simulink model "zad_5_sch_dyskretny"  (R2022b)
settings: Solver=FixedStepAuto  StartTime=0.0  StopTime=1  FixedStep=0.0001  RelTol=1e-3
values from neighbouring files (symbols this model uses):
  A = [0 1 0; a21 0 a23; a31 0 a33]    [zad_5.m]
  B = [0 0; 0 g; b31 0]    [zad_5.m]
  C = [1 0 0]    [zad_5.m]
  Kx = -acker(A, B(:,1), -sKx)    [zad_5.m]
  u0 = -(a31*x1+a33*x3)/b31    [zad_5.m]
  x1 = .003    (= 0.003)    [zad_5.m]
  x2 = 0    [zad_5.m]
  x3 = -(a21*x1+g)/a23    [zad_5.m]
  xd = d-bd    (= 0.0192)    [zad_5.m]
settings Model: Creator=MPatr  LastModifiedBy=AgraWoodAdmin
settings SolverCC: AlgebraicLoopSolver=TrustRegion
settings DebuggingCC: ArithmeticOperatorsInVariantConditions=warning
settings SFSimCC: CustomCodeUndefinedFunction=UseInterfaceOnly

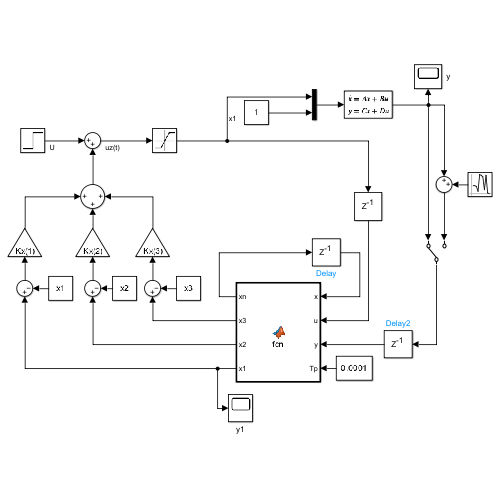
[thumbnail: Simulink's stored preview of the top-level diagram]
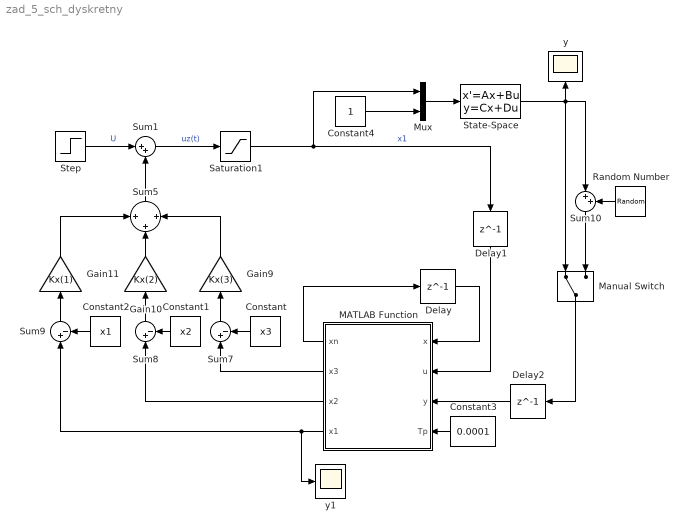
== system zad_5_sch_dyskretny ==
  Constant : Constant  Value=x3
  Constant1 : Constant  Value=x2
  Constant2 : Constant  Value=x1
  Constant3 : Constant  Value=0.0001
  Constant4 : Constant
  Delay : Delay  DelayLength=1  InitialCondition=[xd; 0; 0]
  Delay1 : Delay  DelayLength=1
  Delay2 : Delay  DelayLength=1
  Gain10 : Gain  Gain=Kx(2)
  Gain11 : Gain  Gain=Kx(1)
  Gain9 : Gain  Gain=Kx(3)
  MATLAB Function : MATLAB Function  TreatAsAtomicUnit=on
  Manual Switch : ManualSwitch
  Mux : Mux  Inputs=2
  Random Number : RandomNumber  Variance=.0000001
  Saturation1 : Saturate  UpperLimit=1  LowerLimit=0
  State-Space : StateSpace  A=A  B=B  C=C  D=[0 0]  InitialCondition=[xd; 0; 0]
  Step : Step  Time=0  After=u0  SampleTime=0
  Sum1 : Sum  Inputs=|++
  Sum10 : Sum  Inputs=|++
  Sum5 : Sum  Inputs=+|+|+
  Sum7 : Sum  Inputs=|+-
  Sum8 : Sum  Inputs=|+-
  Sum9 : Sum  Inputs=|+-
  y : Scope
  y1 : Scope
  wires:
  Delay1/1 -> MATLAB Function/2(u)
  Delay2/1 -> MATLAB Function/3(y)
  MATLAB Function/1(xn) -> Delay/1
  Random Number/1 -> Sum10/2
  Manual Switch/1 -> Delay2/1
  Sum10/1 -> Manual Switch/2
  Delay/1 -> MATLAB Function/1(x)
  Constant3/1 -> MATLAB Function/4(Tp)
  Saturation1/1 -> Mux/1, Delay1/1  "x1"
  MATLAB Function/2(x3) -> Sum7/1
  Sum9/1 -> Gain11/1
  MATLAB Function/4(x1) -> y1/1, Sum9/1
  Gain10/1 -> Sum5/2
  Constant/1 -> Sum7/2
  Gain11/1 -> Sum5/1
  Sum8/1 -> Gain10/1
  MATLAB Function/3(x2) -> Sum8/1
  Constant2/1 -> Sum9/2
  Step/1 -> Sum1/1  "U"
  Constant1/1 -> Sum8/2
  Sum7/1 -> Gain9/1
  Sum1/1 -> Saturation1/1  "uz(t)"
  Sum5/1 -> Sum1/2
  Gain9/1 -> Sum5/3
  Mux/1 -> State-Space/1
  Constant4/1 -> Mux/2
  State-Space/1 -> y/1, Sum10/1, Manual Switch/1

== matlab function zad_5_sch_dyskretny/MATLAB Function ==
  data: x input; u input; y input; Tp input; xn output; x3 output; x2 output; x1 output
function [xn, x3, x2, x1]  = fcn(x, u, y, Tp)

m = .00575;
g = 9.81;
FemP1 = .017521;
FemP2 = .0058231;
f1 = .00014142;
f2 = .0045626;
ki = 2.5165;
ci = .0243 * sign(4-2);
d = .0792;
bd = .06;
xd = d-bd;
x10 = .008;
x20 = 0;
x30 = .75;
u10 = 1/ki*(x30-ci);

a21 = 1/(2*m)*x30^2*FemP1/FemP2^2*exp(-x10/FemP2); 
a23 = -1/(m)*x30*FemP1/FemP2*exp(-x10/FemP2); 
a31 = 1/f1*exp(x10/f2)*(ki*u10+ci-x30); 
a33 = -f2/f1*exp(x10/f2);
b31 = ki*f2/f1*exp(x10/f2);
A = [0 1 0; a21 0 a23; a31 0 a33];
B = [0 0; 0 g; b31 0];
C = [1 0 0];
D = 0;

Lo = [413.7108649178256;
      49327.87039995102;
      25.944604383411190];

xnt = (eye(3)+A*Tp)*x + B*Tp*[u; 1] + Lo*Tp*(y-C*x);

xn = xnt(:, 1);
x1 = xn(1);
x2 = xn(2);
x3 = xn(3);
